simulink model "async"  (R2022a)
settings: Solver=FixedStepDiscrete  StartTime=0.0  StopTime=10.0  RelTol=1e-3
libraries: vxlib1 x1
settings Model: Creator=KenYoshioka  LastModifiedBy=KenYoshioka
settings OptimizationCC: DefaultParameterBehavior=Inlined  EnhancedBackFolding=on  PassReuseOutputArgsAs=Individual arguments  ZeroExternalMemoryAtStartup=off  ZeroInternalMemoryAtStartup=off  OptimizeBlockOrder=speed  DifferentSizesBufferReuse=on  OptimizationCustomize=off  EfficientTunableParamExpr=on
settings DebuggingCC: ParameterTunabilityLossMsg=error
settings SFSimCC: MATLABDynamicMemAlloc=off
settings RTWCC: SystemTargetFile=ert.tlc  TemplateMakefile=ert_default_tmf
settings CodeAppCC: ForceParamTrailComments=on  IgnoreCustomStorageClasses=off  OperatorAnnotations=on  SimulinkDataObjDesc=on  SFDataObjDesc=on  InsertBlockDesc=on
settings ERTTargetCC: TargetLangStandard=C99 (ISO)  GenerateSampleERTMain=on  InlinedParameterPlacement=NonHierarchical  ERTCustomFileTemplate=example_file_process.tlc

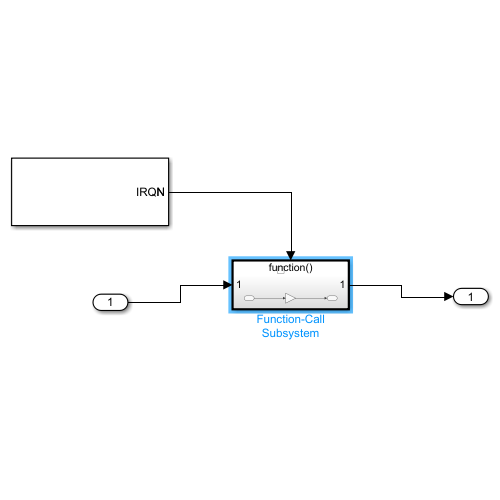
[thumbnail: Simulink's stored preview of the top-level diagram]
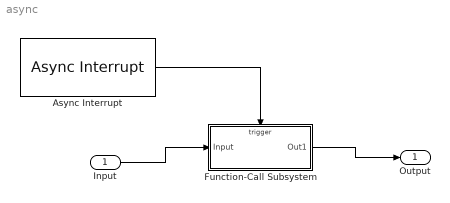
== system async ==
  Input : Inport
  Async Interrupt : vxlib1/Async Interrupt  irqnumbers=[1 2]  irqoffsets=[192 193]  irqpriorities=[10 11]  irqpreempts=[0 1]  manageowntimer=on  tickres=1/60  ticklen=32bits  showinput=off
      settings: SourceProductBaseCode=SL
  Function-Call Subsystem : Subsystem  TreatAsAtomicUnit=on
  Output : Outport
  wires:
  Async Interrupt/1 -> Function-Call Subsystem/Trigger
  Input/1 -> Function-Call Subsystem/1(Input)
  Function-Call Subsystem/1(Out1) -> Output/1

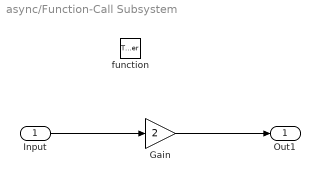
== system async/Function-Call Subsystem ==
  Input : Inport
  function : TriggerPort  TriggerType=function-call  VariantControl=(inherit)
  Gain : Gain  Gain=2
  Out1 : Outport
  wires:
  Input/1 -> Gain/1
  Gain/1 -> Out1/1
